simulink model "Problem3"  (R2020a)
settings: Solver=ode45  StartTime=0.0  StopTime=10  RelTol=1e-3
model workspace (MAT data in the model file):
  Ki = -32.306
  Kp = -274.3608
  Ts = 0
  b = 50
  m = 1000
  u = 500
settings Model: OrderedModelArguments=off  Creator=tanu  LastModifiedBy=tanu
settings DebuggingCC: ModelReferenceExtraNoncontSigs=none

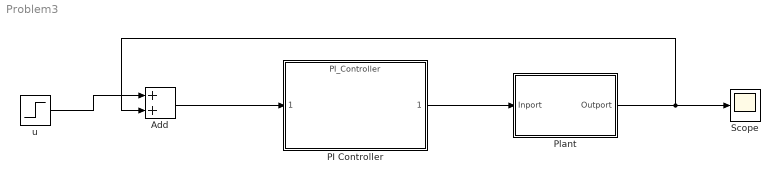
== system Problem3 ==
  Add : Sum
  PI Controller : ModelReference  ModelNameDialog=PI_Controller  SimulationMode=Normal  ModelReferenceVersion=1.9
  Plant : Subsystem
  Scope : Scope
  u : Step  Time=0  After=10  SampleTime=0
  wires:
  Plant/1(Outport) -> Scope/1, Add/2
  u/1 -> Add/1
  Add/1 -> PI Controller/1
  PI Controller/1 -> Plant/1(Inport)

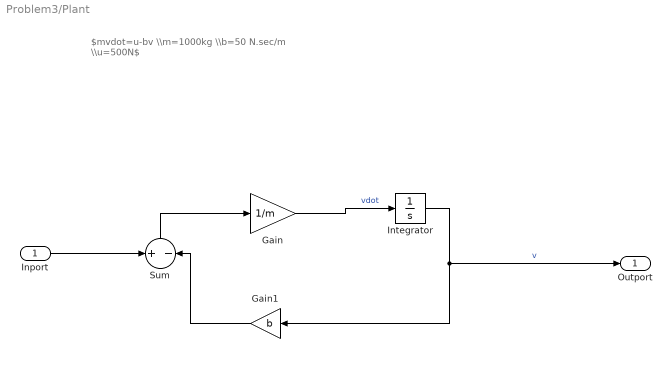
== system Problem3/Plant ==
  note: $mvdot=u-bv \\m=1000kg \\b=50 N.sec/m \\u=500N$
  Inport : Inport
  Gain : Gain  Gain=1/m
  Gain1 : Gain  Gain=b
  Integrator : Integrator
  Sum : Sum  Inputs=+-
  Outport : Outport
  wires:
  Integrator/1 -> Outport/1, Gain1/1  "v"
  Sum/1 -> Gain/1
  Gain/1 -> Integrator/1  "vdot"
  Inport/1 -> Sum/1
  Gain1/1 -> Sum/2
